simulink model "speed"  (R2023b)
settings: Solver=VariableStepAuto  StartTime=0.0  StopTime=0.1  RelTol=1e-3
settings Model: Creator=George  LastModifiedBy=volko

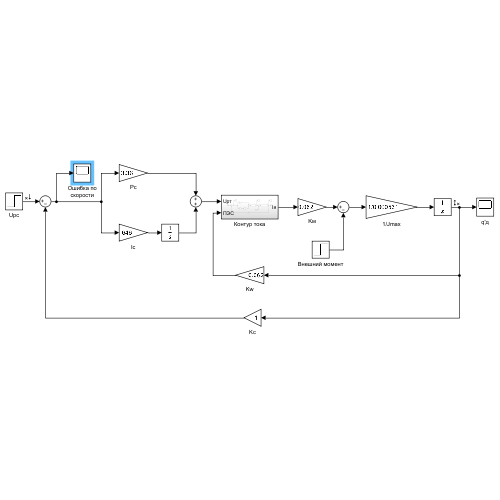
[thumbnail: Simulink's stored preview of the top-level diagram]
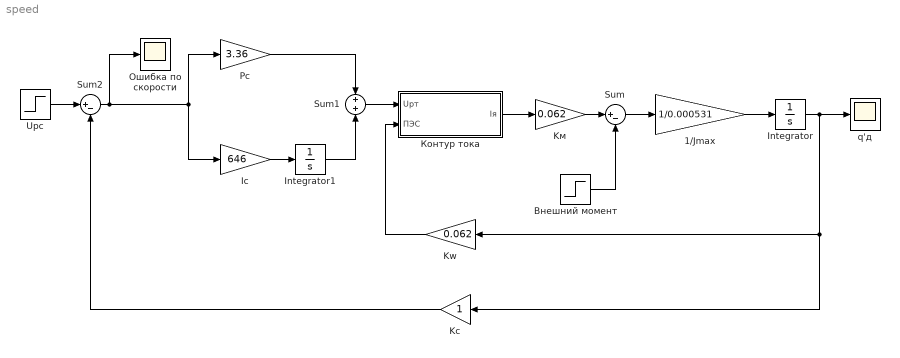
== system speed ==
  1/Jmax : Gain  Gain=1/0.000531
  Integrator : Integrator
  Integrator1 : Integrator
  Iс : Gain  Gain=646
  Kw : Gain  Gain=0.062
  Kм : Gain  Gain=0.062
  Kс : Gain
  Pс : Gain  Gain=3.36
  Sum : Sum  Inputs=|+-
  Sum1 : Sum
  Sum2 : Sum  Inputs=|+-
  Uрс : Step  Time=0  SampleTime=0
  q'д : Scope
  Внешний момент : Step  Time=0.05  After=0.47  SampleTime=0
  Контур тока : Subsystem
  Ошибка по скорости : Scope
  wires:
  Kw/1 -> Контур тока/2(ПЭС)
  Контур тока/1(Iя) -> Kм/1
  Внешний момент/1 -> Sum/2
  Kм/1 -> Sum/1
  Sum/1 -> 1/Jmax/1
  1/Jmax/1 -> Integrator/1
  Integrator/1 -> Kс/1, Kw/1, q'д/1
  Integrator1/1 -> Sum1/2
  Sum1/1 -> Контур тока/1(Uрт)
  Sum2/1 -> Ошибка по скорости/1, Pс/1, Iс/1
  Kс/1 -> Sum2/2
  Uрс/1 -> Sum2/1
  Iс/1 -> Integrator1/1
  Pс/1 -> Sum1/1

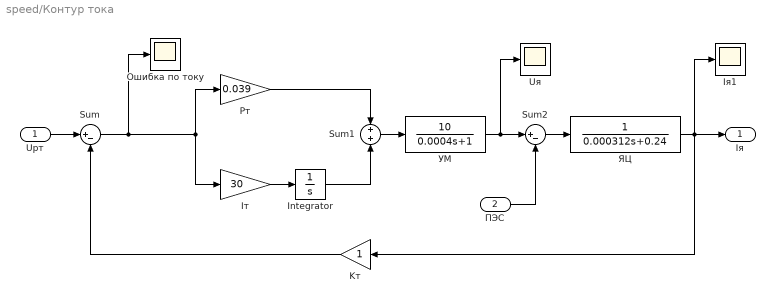
== system speed/Контур тока ==
  Uрт : Inport
  ПЭС : Inport  Port=2
  Integrator : Integrator
  Iт : Gain  Gain=30
  Iя1 : Scope
  Kт : Gain
  Pт : Gain  Gain=0.039
  Sum : Sum  Inputs=|+-
  Sum1 : Sum
  Sum2 : Sum  Inputs=|+-
  Uя : Scope
  Ошибка по току : Scope
  УМ : TransferFcn  Numerator=[10]  Denominator=[0.0004 1]
  ЯЦ : TransferFcn  Denominator=[0.000312 0.24]
  Iя : Outport
  wires:
  УМ/1 -> Sum2/1, Uя/1
  Integrator/1 -> Sum1/2
  Sum1/1 -> УМ/1
  Iт/1 -> Integrator/1
  Sum/1 -> Ошибка по току/1, Iт/1, Pт/1
  ЯЦ/1 -> Iя1/1, Iя/1, Kт/1
  Kт/1 -> Sum/2
  Pт/1 -> Sum1/1
  Uрт/1 -> Sum/1
  Sum2/1 -> ЯЦ/1
  ПЭС/1 -> Sum2/2
